simulink model "PWM"  (R2022b)
settings: Solver=VariableStepAuto  StartTime=0.0  StopTime=0.001  RelTol=1e-3
libraries: spspowerguiLib x1
settings Model: Creator=Biplov Jha  LastModifiedBy=Biplov Jha

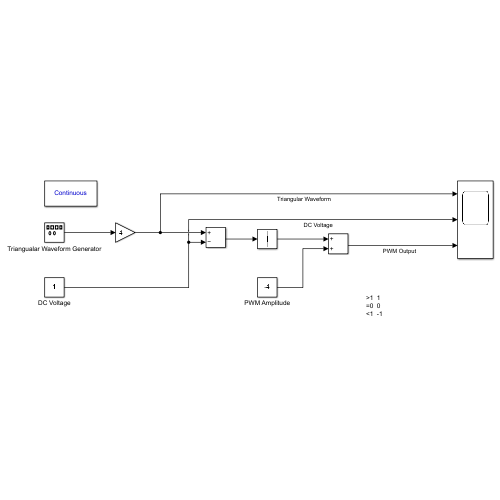
[thumbnail: Simulink's stored preview of the top-level diagram]
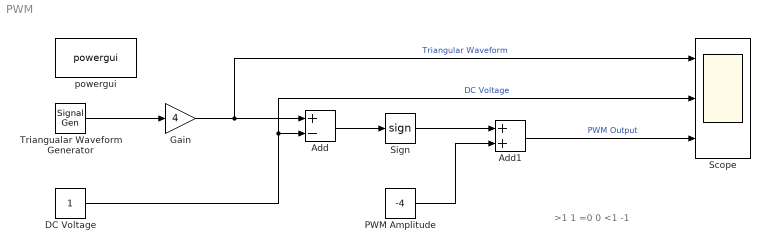
== system PWM ==
  note: >1  1
      | =0  0
      | <1  -1
  Add : Sum  Inputs=+-
  Add1 : Sum
  DC Voltage : Constant
  Gain : Gain  Gain=4
  PWM Amplitude : Constant  Value=-4
  Scope : Scope  NumInputPorts=3
  Sign : Signum
  Triangualar Waveform Generator : SignalGenerator  WaveForm=sawtooth  Frequency=25e3
  powergui : spspowerguiLib/powergui  Priority=1  SimulationMode=Continuous  SampleTime=50e-6  frequency=60  Iterations=50  frequencyindice=60  Pbase=100e6  ErrMax=1e-4  UnitsV=kV  UnitsW=MW  buscounter=0  FunctionMessages=off  echomessages=off  EnableUseOfTLC=off  CurrentSourceSwitches=off  DisableSnubberDevices=off  DisableRonSwitches=off  DisableVfSwitches=off  DisplayEquations=off  AutomaticDiscreteSolvers=off  SolverType=Tustin/Backward Euler (TBE)  Interpol=off  ExternalGateDelay=off  methode=off  Ts=100  x0status=blocks  SPID=on  SwTol=0  HookPort=off  NonlinearTolerance=1e-4  nMaxIteration=100  ContinueOnMaxIteration=off  RestoreLinks=warning  ResistiveCurrentMeasurement=off  Frange=[0:2:500]  Ylog=off  Xlog=on  ShowGrid=off  save=off  variable=ZData  structure=0  ZoomFFT=off  StartTime=0.0  cycles=1  DisplayStyle=1  fundamental=60  FreqAxis=off  MaxFrequency=1000  frequencyindicesteady=1  RmsSteady=1  display=off
  wires:
  Triangualar Waveform Generator/1 -> Gain/1
  Gain/1 -> Scope/1, Add/1  "Triangular Waveform"
  DC Voltage/1 -> Scope/2, Add/2  "DC Voltage"
  Add/1 -> Sign/1
  Sign/1 -> Add1/1
  PWM Amplitude/1 -> Add1/2
  Add1/1 -> Scope/3  "PWM Output"
